simulink model "Group44PACEMAKER"  (R2022b)
settings: Solver=FixedStepAuto  StartTime=0.0  StopTime=2  FixedStep=1e-2  RelTol=1e-3  EnableMultiTasking=on
undefined symbols (not defined in the file): D0, D1, D10, D11, D12, D13, D2, D3, D4, D5, D6, D7, D8, D9, PTA0, PTA1, PTA2, PTB23, PTB9, PTC16, PTC17, PTC2, PTC3, PTC4, PTD0, PTD1, PTD2, PTD3
libraries: frdmk64flib x15, dsparch4 x1, dspstat3 x1
(part 2 of 2)

== stateflow chart Group44PACEMAKER/Stateflow/Chart ==
  state PaceAtria
    entry:
    %Closes proper switches to pace the atrium
    PACE_CHARGE_CTRL = false;
    PACE_GND_CTRL = true;
    ATR_PACE_CTRL = true;
    ATR_GND_CTRL = false;
    Z_ATR_CTRL = false;
    Z_VENT_CTRL = false;
    VENT_GND_CTRL = false;
    VENT_PACE_CTRL = false;
  state Collector_State
    %All modes lead back to here
  state PaceVentricle
    entry:
    %Closes proper switches to pace the ventricle
    PACE_CHARGE_CTRL = false;
    PACE_GND_CTRL = true;
    ATR_PACE_CTRL = false;
    ATR_GND_CTRL = false;
    Z_ATR_CTRL = false;
    Z_VENT_CTRL = false;
    VENT_GND_CTRL = false;
    VENT_PACE_CTRL = true;
  state ChargeC22_Ventricular_DischargeC21
    entry:
    %This state charges C22 to pace the heart and discharges C21 through the ventricle
    ATR_PACE_CTRL = false;
    VENT_PACE_CTRL = false;
    PACE_CHARGE_CTRL = true;
    PACE_GND_CTRL = true;
    Z_ATR_CTRL = false;
    Z_VENT_CTRL = false;
    ATR_GND_CTRL = false;
    VENT_GND_CTRL = true;
  state ChargeC22_Atrial_DischargeC21
    entry:
    %This state charges C22 to pace the heart and discharges C21 through the atrium
    ATR_PACE_CTRL = false;
    VENT_PACE_CTRL = false;
    PACE_CHARGE_CTRL = true;
    PACE_GND_CTRL = true;
    Z_ATR_CTRL = false;
    Z_VENT_CTRL = false;
    ATR_GND_CTRL = true;
    VENT_GND_CTRL = false;
  state Initial_State
    %This is where we will set parameters that will stay constant throughout the stateflow
    in_default = true;
  state VentricularAlertPeriod
    entry:
    %Closes the frontend control to allow the pacemaker to sense the heart
    %Frontend gets opened once you leave this state
    FRONTEND_CTRL = true;
    exit:
    FRONTEND_CTRL = false;
  state AtrialAlertPeriod
    entry:
    %Closes the frontend control to allow the pacemaker to sense the heart
    %Frontend gets opened once you leave this state
    FRONTEND_CTRL = true;
    exit:
    FRONTEND_CTRL = false;
  PaceVentricle -> Collector_State : after(vPulseWidth,msec)
  PaceAtria -> Collector_State : after(aPulseWidth,msec)
  ChargeC22_Atrial_DischargeC21 -> Collector_State [order 2] : [mode~="AOO" && mode~="AAI"]
  ChargeC22_Ventricular_DischargeC21 -> Collector_State [order 1] : [mode~="VOO" && mode~="VVI"]
  Collector_State -> (junction 127)
  (junction 144) -> PaceAtria [order 2] : after(LRL-aPulseWidth,msec)[mode=="AOO"]
  (junction 143) -> PaceVentricle [order 2] : after(LRL-vPulseWidth,msec)[mode=="VOO"]
  AtrialAlertPeriod -> PaceAtria [order 2] : after(LRL-ARP-aPulseWidth,msec)
  VentricularAlertPeriod -> PaceVentricle [order 2] : after(LRL-VRP-vPulseWidth,msec)
  ChargeC22_Ventricular_DischargeC21 -> (junction 143) [order 2]
  ChargeC22_Atrial_DischargeC21 -> (junction 144) [order 1]
  (junction 127) -> ChargeC22_Atrial_DischargeC21 [order 2] : [mode=="AOO"||mode=="AAI"]{pulseDutyCycle=aPulseAmp/5.0*100}
  (junction 127) -> ChargeC22_Ventricular_DischargeC21 [order 1] : [mode=="VOO"||mode=="VVI"]{pulseDutyCycle=vPulseAmp/5.0*100}
  (junction 143) -> VentricularAlertPeriod [order 1] : after(VRP,msec)[mode=="VVI"]{cmpDutyCycle=vSensitivity/5.0*100}
  Initial_State -> (junction 127) : {in_default = false}
  (junction 144) -> AtrialAlertPeriod [order 1] : after(ARP,msec)[mode=="AAI"]{cmpDutyCycle=aSensitivity/5.0*100}
  AtrialAlertPeriod -> ChargeC22_Atrial_DischargeC21 [order 1] : [ATR_CMP_DETECT == true ]
  VentricularAlertPeriod -> ChargeC22_Ventricular_DischargeC21 [order 1] : [VENT_CMP_DETECT == true ]
  (default) -> Initial_State
  data: mode input; ARP input; VRP input; aPulseWidth input; aPulseAmp input; vPulseWidth input; vPulseAmp input; aSensitivity input; vSensitivity input; LRL input; ATR_CMP_DETECT input; VENT_CMP_DETECT input; ATR_GND_CTRL output; ATR_PACE_CTRL output; FRONTEND_CTRL output; PACE_CHARGE_CTRL output; PACE_GND_CTRL output; VENT_GND_CTRL output; VENT_PACE_CTRL output; Z_ATR_CTRL output; Z_VENT_CTRL output; cmpDutyCycle output; in_default output; pulseDutyCycle output
